simulink model "SendToTcpServer"  (R2018b)
settings: Solver=FixedStepAuto  StartTime=0.0  StopTime=inf  RelTol=1e-3  EnableMultiTasking=on
libraries: arduinowifilib x1
settings Model: SimulationMode=external  ExtModeTrigDuration=2  Creator=Gerard  LastModifiedBy=Gerard
settings OptimizationCC: EnhancedBackFolding=on  PassReuseOutputArgsAs=Individual arguments  MaxStackSize=64  OptimizeBlockOrder=speed  DifferentSizesBufferReuse=on  OptimizationCustomize=off
settings DebuggingCC: ParameterTunabilityLossMsg=error
settings HardwareCC: ProdBitPerPointer=32  ProdBitPerSizeT=32  ProdBitPerPtrDiffT=32  ProdLargestAtomicInteger=Long  ProdLargestAtomicFloat=Double  ProdWordSize=32  ProdHWDeviceType=ARM Compatible->ARM Cortex  UseEmbeddedCoderFeatures=off  UseSimulinkCoderFeatures=off
settings SFSimCC: MATLABDynamicMemAlloc=off
settings RTWCC: SystemTargetFile=ert.tlc  HardwareBoard=Arduino MKR1000  TemplateMakefile=ert_default_tmf  GenerateReport=on  Toolchain=Arduino ARM  BuildConfiguration=Faster Runs  IncludeHyperlinkInReport=on  LaunchReport=on  GenerateTraceInfo=on  GenerateTraceReport=on  GenerateTraceReportSl=on  GenerateTraceReportSf=on  GenerateTraceReportEml=on
settings CodeAppCC: ForceParamTrailComments=on  IgnoreCustomStorageClasses=off  OperatorAnnotations=on  SimulinkDataObjDesc=on  SFDataObjDesc=on  InsertBlockDesc=on
settings ERTTargetCC: SupportContinuousTime=on  SupportNonInlinedSFcns=on  SupportVariableSizeSignals=on

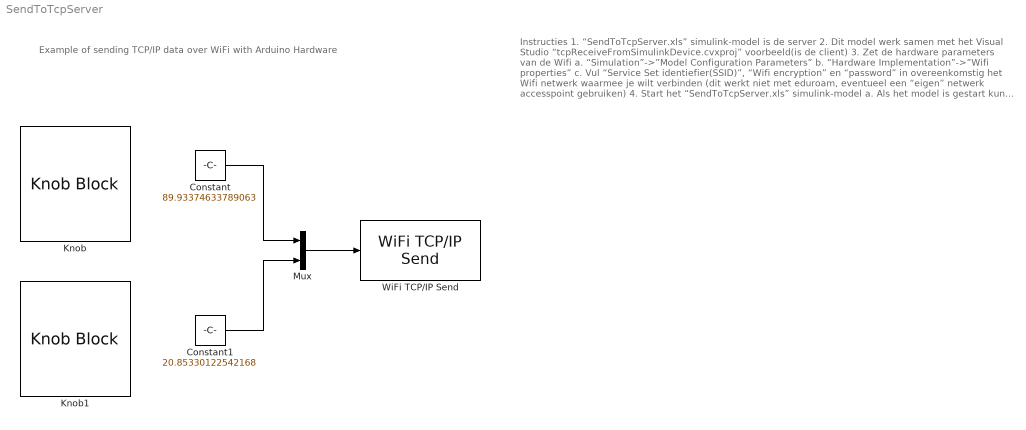
== system SendToTcpServer ==
  note: Example of sending TCP/IP data over WiFi
      | with Arduino Hardware
  note: Instructies
      | 1. “SendToTcpServer.xls” simulink-model is de server
      | 2. Dit model werk samen met het Visual Studio “tcpReceiveFromSimulinkDevice.cvxproj” voorbeeld(is de client)
      | 3. Zet de hardware parameters van de Wifi
      | a. “Simulation”->”Model Configuration Parameters”
      | b. “Hardware Implementation”->”Wifi properties”
      | c. Vul “Service Set identiefier(SSID)”, “Wifi encryption” en “password” in overeenkomstig het Wifi netwerk waarmee je wilt verbinden (dit werkt niet met eduroam, eventueel een “eigen” netwerk accesspoint gebruiken)
      | 4. Start het “SendToTcpServer.xls” simulink-model
      | a. Als het model is gestart kun je zien wel ip-address er aan het model is toegewezen door het accesspoint, click het “View diagnostics” item onderaan het model(alleen zichtbaar al het model in running is)
      | 5. Vul het ip-address van de server in het bestand “tcpReceiveFromSimulinkDevice.cpp” in op de regel van “#define IP_ADDRESS "192.168.2.87"
      | 6. Start "tcpReceiveFromSimulinkDevice.cvxproj" Visual Studio project
      | Auteur: Gerard Harkema
      | Versie: 1.0
      | Datum: 6 april 2019
  Constant : Constant  Value=89.93374633789063  OutDataTypeStr=double
  Constant1 : Constant  Value=20.85330122542168  OutDataTypeStr=double
  Knob : KnobBlock  WebBlockId=22
  Knob1 : KnobBlock  WebBlockId=23
  Mux : Mux  Inputs=2
  WiFi TCP/IP Send : arduinowifilib/WiFi TCP//IP Send  Mode_=Server  serverport=25000  RemoteAddr_=192.168.1.2  RemoteServerPort_=25000  remoteipoctet1=192  remoteipoctet2=168  remoteipoctet3=1  remoteipoctet4=2  wifiTCPServerIndex=0  wifiTCPClientIndex=0  blockPlatform=ARDUINO  isARMArch=true  SimulateUsing=Code generation
      settings: SourceProductName=Simulink Support Package for Arduino Hardware  SourceProductBaseCode=ARDUINO
  wires:
  Constant/1 -> Mux/1
  Constant1/1 -> Mux/2
  Mux/1 -> WiFi TCP/IP Send/1
